simulink model "GS_model"  (R2018b)
settings: Solver=ode5  StartTime=0.0  StopTime=SimuStopTime  FixedStep=T_Simu  RelTol=1e-3
InitFcn:
  | Initial
undefined symbols (not defined in the file or in its folder): Aba10, Aba20, aeroCIP2006_S, aeroCIP2006_X, aeroCIP2006_Y, Agl0, Ass_kS, Ass_n1, Ass_n2, Ass_n3, Ass_n4, Ass_Noise, Ass_R, Ass_Resolution, Ass_TmOrder, AssA_Fix_Abs, AssB_Fix_Abs, AssC_Fix_Abs, AssD_Fix_Abs, AssE_Fix_Aps, AssF_Fix_Aps, C, c_max, c_min, Cd, CenterOfFigNX, CenterOfFigNY, CenterOfFigNZ, CenterOfFigP1, CenterOfFigP2, CenterOfFigPX, CenterOfFigPY, CenterOfFigPZ, Cmu, Crou, DEG2RAD, DiscIntNeverNeededParam, Eg_Dir, Eg_F, Eg_PrepareTime, Eg_r_L_L, Fw_Abf, Fw_Hmax, Fw_J, Fw_Spd0, Fw_Tmax, git_hash_BaseLine, git_hash_Project, Gnss_Noise_Pos, Gnss_Noise_Vel, Gnss_PropgationTime, GyroA_Fix_Abg, GyroA_Noise, GyroB_Fix_Abg, GyroB_Noise, GyroC_Fix_Abg, GyroC_Noise, GyroD_Fix_Abg, GyroD_Noise, h ... (+94)
libraries: simulink x308, sharedutil x46, aerolibutil x37, sharedtransform x31, vrlib x14, aerolibgravity2 x2
(part 8 of 20)

== system GS_model/Subsystem2/Subsystem/Sensor/Magnetometer/MmModel1/Mm_ErrSet ==
  note: TC_MmGNDSet[5*1]
  note: TC_MmErr_Constant[3*1]
  note: TC_MmErr_WildValue[3*1]
  note: TC_MmErr_Jump[5*1]
  note: TC_MmErr_Wave[4*1]
  Mm_MagneticIntensity : Inport
  Mm_Num : Inport  Port=2
  TC_Mm : Inport  Port=3
  Constant1 : Constant  Value=0
  Constant2 : Constant  Value=0
  Demux : Demux  Outputs=[5;3;5;4;3]
  Demux1 : Demux  Outputs=[1;4]
  Demux10 : Demux  Outputs=[1;2]
  Demux6 : Demux  Outputs=[1;2]
  Demux7 : Demux  Outputs=[1;4]
  Demux8 : Demux  Outputs=[1;3]
  Demux9 : Demux  Outputs=[1;3]
  If Action Subsystem3 : Subsystem  TreatAsAtomicUnit=on
  If Action Subsystem4 : Subsystem  TreatAsAtomicUnit=on
  If1 : If  IfExpression=u1 == 1
  Logical Operator{1..5} (5 alike) : Logic  Operator=OR  AllPortsSameDT=off  OutDataTypeStr=boolean
  Merge1 : Merge
  MmErrSet : Subsystem
  Relational Operator{1..10} (10 alike) : RelationalOperator  Operator===  OutDataTypeStr=boolean  RndMeth=Simplest
  Triggered Subsystem5 : Subsystem  TreatAsAtomicUnit=on
  Triggered Subsystem6 : Subsystem  TreatAsAtomicUnit=on
  Triggered Subsystem7 : Subsystem  TreatAsAtomicUnit=on
  Triggered Subsystem8 : Subsystem  TreatAsAtomicUnit=on
  Triggered Subsystem9 : Subsystem  TreatAsAtomicUnit=on
  TM_Mm : Outport
  wires:
  TC_Mm/1 -> Demux/1
  Demux/1 -> Demux1/1
  Demux/2 -> Demux6/1
  Demux/3 -> Demux7/1
  Demux/4 -> Demux9/1
  Demux/5 -> Demux10/1
  Demux1/1 -> Relational Operator1/2, Relational Operator5/2
  Demux1/2 -> Triggered Subsystem6/1(In1)
  Triggered Subsystem6/1(Out1) -> Demux8/1
  Demux8/1 -> If1/1
  If1/1 -> If Action Subsystem4/Action
  Demux8/2 -> If Action Subsystem4/1(In1)
  If Action Subsystem4/1(Out1) -> Merge1/1
  MmErrSet/1(Mm_out) -> If Action Subsystem3/1(In1)
  If1/2 -> If Action Subsystem3/Action
  If Action Subsystem3/1(Out1) -> Merge1/2
  Mm_MagneticIntensity/1 -> MmErrSet/1(Mm_MagneticIntensity)
  Triggered Subsystem9/1(Out1) -> MmErrSet/2(TC_MmErrSet_Constant)
  Triggered Subsystem5/1(Out1) -> MmErrSet/3(TC_MmErrSet_Jump)
  Triggered Subsystem7/1(Out1) -> MmErrSet/4(TC_MmErrSet_Wave)
  Triggered Subsystem8/1(Out1) -> MmErrSet/5(TC_MmErrSet_WildValue)
  Merge1/1 -> TM_Mm/1
  Relational Operator10/1 -> Logical Operator4/1
  Logical Operator4/1 -> Triggered Subsystem8/Enable
  Relational Operator3/1 -> Logical Operator2/1
  Relational Operator6/1 -> Logical Operator1/2
  Demux7/1 -> Relational Operator3/2, Relational Operator7/2
  Mm_Num/1 -> Relational Operator9/1, Relational Operator8/1, Relational Operator7/1, Relational Operator6/1, Relational Operator5/1
  Logical Operator2/1 -> Triggered Subsystem5/Enable
  Relational Operator7/1 -> Logical Operator2/2
  Relational Operator9/1 -> Logical Operator4/2
  Relational Operator4/1 -> Logical Operator3/1
  Logical Operator3/1 -> Triggered Subsystem7/Enable
  Relational Operator8/1 -> Logical Operator3/2
  Demux10/1 -> Relational Operator10/2, Relational Operator9/2
  Relational Operator2/1 -> Logical Operator1/1
  Logical Operator1/1 -> Triggered Subsystem9/Enable
  Demux6/1 -> Relational Operator2/2, Relational Operator6/2
  Constant2/1 -> Relational Operator10/1, Relational Operator4/1, Relational Operator3/1, Relational Operator2/1
  Demux9/1 -> Relational Operator4/2, Relational Operator8/2
  Demux10/2 -> Triggered Subsystem8/1(In1)
  Demux9/2 -> Triggered Subsystem7/1(In1)
  Demux7/2 -> Triggered Subsystem5/1(In1)
  Demux6/2 -> Triggered Subsystem9/1(In1)
  Relational Operator5/1 -> Logical Operator5/2
  Constant1/1 -> Relational Operator1/1
  Relational Operator1/1 -> Logical Operator5/1
  Logical Operator5/1 -> Triggered Subsystem6/Enable

== system GS_model/Subsystem2/Subsystem/Sensor/Magnetometer/MmModel1/Mm_MathModel ==
  Bb : Inport
  Mm_Fix_Abm : Inport  Port=2
  Mm_MtInflunce_Coff : Inport  Port=3
  Mm_Noise : Inport  Port=4
  M_Mt : Inport  Port=5
  Math Function : Math  Operator=transpose  SaturateOnIntegerOverflow=on
  Product1 : Product  Multiplication=Matrix(*)  RndMeth=Zero
  Product2 : Product  Multiplication=Matrix(*)  RndMeth=Zero
  Sum1 : Sum  Inputs=|++
  Sum2 : Sum  Inputs=|++
  Mm_MagneticIntensity : Outport
  wires:
  M_Mt/1 -> Product1/2
  Mm_Noise/1 -> Sum1/2
  Product1/1 -> Sum2/2
  Sum1/1 -> Mm_MagneticIntensity/1
  Mm_Fix_Abm/1 -> Math Function/1
  Mm_MtInflunce_Coff/1 -> Product1/1
  Math Function/1 -> Product2/1
  Bb/1 -> Product2/2
  Sum2/1 -> Sum1/1
  Product2/1 -> Sum2/1

== system GS_model/Subsystem2/Subsystem/Sensor/Magnetometer/MmModel2/Mm_ErrSet ==
  note: TC_MmErr_Wave[4*1]
  note: TC_MmErr_Jump[5*1]
  note: TC_MmErr_WildValue[3*1]
  note: TC_MmErr_Constant[3*1]
  note: TC_MmGNDSet[5*1]
  Mm_MagneticIntensity : Inport
  Mm_Num : Inport  Port=2
  TC_Mm : Inport  Port=3
  Constant1 : Constant  Value=0
  Constant2 : Constant  Value=0
  Demux : Demux  Outputs=[5;3;5;4;3]
  Demux1 : Demux  Outputs=[1;4]
  Demux10 : Demux  Outputs=[1;2]
  Demux6 : Demux  Outputs=[1;2]
  Demux7 : Demux  Outputs=[1;4]
  Demux8 : Demux  Outputs=[1;3]
  Demux9 : Demux  Outputs=[1;3]
  If Action Subsystem3 : Subsystem  TreatAsAtomicUnit=on
  If Action Subsystem4 : Subsystem  TreatAsAtomicUnit=on
  If1 : If  IfExpression=u1 == 1
  Logical Operator{1..5} (5 alike) : Logic  Operator=OR  AllPortsSameDT=off  OutDataTypeStr=boolean
  Merge1 : Merge
  MmErrSet : Subsystem
  Relational Operator{1..10} (10 alike) : RelationalOperator  Operator===  OutDataTypeStr=boolean  RndMeth=Simplest
  Triggered Subsystem5 : Subsystem  TreatAsAtomicUnit=on
  Triggered Subsystem6 : Subsystem  TreatAsAtomicUnit=on
  Triggered Subsystem7 : Subsystem  TreatAsAtomicUnit=on
  Triggered Subsystem8 : Subsystem  TreatAsAtomicUnit=on
  Triggered Subsystem9 : Subsystem  TreatAsAtomicUnit=on
  TM_Mm : Outport
  wires:
  Logical Operator5/1 -> Triggered Subsystem6/Enable
  Relational Operator1/1 -> Logical Operator5/1
  Constant1/1 -> Relational Operator1/1
  Relational Operator5/1 -> Logical Operator5/2
  Demux6/2 -> Triggered Subsystem9/1(In1)
  Demux7/2 -> Triggered Subsystem5/1(In1)
  Demux9/2 -> Triggered Subsystem7/1(In1)
  Demux10/2 -> Triggered Subsystem8/1(In1)
  Demux9/1 -> Relational Operator8/2, Relational Operator4/2
  Constant2/1 -> Relational Operator2/1, Relational Operator3/1, Relational Operator4/1, Relational Operator10/1
  Demux6/1 -> Relational Operator6/2, Relational Operator2/2
  Logical Operator1/1 -> Triggered Subsystem9/Enable
  Relational Operator2/1 -> Logical Operator1/1
  Demux10/1 -> Relational Operator9/2, Relational Operator10/2
  Relational Operator8/1 -> Logical Operator3/2
  Logical Operator3/1 -> Triggered Subsystem7/Enable
  Relational Operator4/1 -> Logical Operator3/1
  Relational Operator9/1 -> Logical Operator4/2
  Relational Operator7/1 -> Logical Operator2/2
  Logical Operator2/1 -> Triggered Subsystem5/Enable
  Mm_Num/1 -> Relational Operator5/1, Relational Operator6/1, Relational Operator7/1, Relational Operator8/1, Relational Operator9/1
  Demux7/1 -> Relational Operator7/2, Relational Operator3/2
  Relational Operator6/1 -> Logical Operator1/2
  Relational Operator3/1 -> Logical Operator2/1
  Logical Operator4/1 -> Triggered Subsystem8/Enable
  Relational Operator10/1 -> Logical Operator4/1
  Merge1/1 -> TM_Mm/1
  Triggered Subsystem8/1(Out1) -> MmErrSet/5(TC_MmErrSet_WildValue)
  Triggered Subsystem7/1(Out1) -> MmErrSet/4(TC_MmErrSet_Wave)
  Triggered Subsystem5/1(Out1) -> MmErrSet/3(TC_MmErrSet_Jump)
  Triggered Subsystem9/1(Out1) -> MmErrSet/2(TC_MmErrSet_Constant)
  Mm_MagneticIntensity/1 -> MmErrSet/1(Mm_MagneticIntensity)
  If Action Subsystem3/1(Out1) -> Merge1/2
  If1/2 -> If Action Subsystem3/Action
  MmErrSet/1(Mm_out) -> If Action Subsystem3/1(In1)
  If Action Subsystem4/1(Out1) -> Merge1/1
  Demux8/2 -> If Action Subsystem4/1(In1)
  If1/1 -> If Action Subsystem4/Action
  Demux8/1 -> If1/1
  Triggered Subsystem6/1(Out1) -> Demux8/1
  Demux1/2 -> Triggered Subsystem6/1(In1)
  Demux1/1 -> Relational Operator5/2, Relational Operator1/2
  Demux/5 -> Demux10/1
  Demux/4 -> Demux9/1
  Demux/3 -> Demux7/1
  Demux/2 -> Demux6/1
  Demux/1 -> Demux1/1
  TC_Mm/1 -> Demux/1

== system GS_model/Subsystem2/Subsystem/Sensor/Magnetometer/MmModel2/Mm_MathModel ==
  Bb : Inport
  Mm_Fix_Abm : Inport  Port=2
  Mm_MtInflunce_Coff : Inport  Port=3
  Mm_Noise : Inport  Port=4
  MtCoff : Inport  Port=5
  Math Function : Math  Operator=transpose  SaturateOnIntegerOverflow=on
  Product1 : Product  Multiplication=Matrix(*)  RndMeth=Zero
  Product2 : Product  Multiplication=Matrix(*)  RndMeth=Zero
  Sum1 : Sum  Inputs=|++
  Sum2 : Sum  Inputs=|++
  Mm_MagneticIntensity : Outport
  wires:
  Product2/1 -> Sum2/1
  Sum2/1 -> Sum1/1
  Bb/1 -> Product2/2
  Math Function/1 -> Product2/1
  Mm_MtInflunce_Coff/1 -> Product1/1
  Mm_Fix_Abm/1 -> Math Function/1
  Sum1/1 -> Mm_MagneticIntensity/1
  Product1/1 -> Sum2/2
  Mm_Noise/1 -> Sum1/2
  MtCoff/1 -> Product1/2

== system GS_model/Subsystem2/Subsystem/Sensor/Magnetometer/MmModel3/Mm_ErrSet ==
  note: TC_MmGNDSet[5*1]
  note: TC_MmErr_Constant[3*1]
  note: TC_MmErr_WildValue[3*1]
  note: TC_MmErr_Jump[5*1]
  note: TC_MmErr_Wave[4*1]
  Mm_MagneticIntensity : Inport
  Mm_Num : Inport  Port=2
  TC_Mm : Inport  Port=3
  Constant1 : Constant  Value=0
  Constant2 : Constant  Value=0
  Demux : Demux  Outputs=[5;3;5;4;3]
  Demux1 : Demux  Outputs=[1;4]
  Demux10 : Demux  Outputs=[1;2]
  Demux6 : Demux  Outputs=[1;2]
  Demux7 : Demux  Outputs=[1;4]
  Demux8 : Demux  Outputs=[1;3]
  Demux9 : Demux  Outputs=[1;3]
  If Action Subsystem3 : Subsystem  TreatAsAtomicUnit=on
  If Action Subsystem4 : Subsystem  TreatAsAtomicUnit=on
  If1 : If  IfExpression=u1 == 1
  Logical Operator{1..5} (5 alike) : Logic  Operator=OR  AllPortsSameDT=off  OutDataTypeStr=boolean
  Merge1 : Merge
  MmErrSet : Subsystem
  Relational Operator{1..10} (10 alike) : RelationalOperator  Operator===  OutDataTypeStr=boolean  RndMeth=Simplest
  Triggered Subsystem5 : Subsystem  TreatAsAtomicUnit=on
  Triggered Subsystem6 : Subsystem  TreatAsAtomicUnit=on
  Triggered Subsystem7 : Subsystem  TreatAsAtomicUnit=on
  Triggered Subsystem8 : Subsystem  TreatAsAtomicUnit=on
  Triggered Subsystem9 : Subsystem  TreatAsAtomicUnit=on
  TM_Mm : Outport
  wires:
  TC_Mm/1 -> Demux/1
  Demux/1 -> Demux1/1
  Demux/2 -> Demux6/1
  Demux/3 -> Demux7/1
  Demux/4 -> Demux9/1
  Demux/5 -> Demux10/1
  Demux1/1 -> Relational Operator1/2, Relational Operator5/2
  Demux1/2 -> Triggered Subsystem6/1(In1)
  Triggered Subsystem6/1(Out1) -> Demux8/1
  Demux8/1 -> If1/1
  If1/1 -> If Action Subsystem4/Action
  Demux8/2 -> If Action Subsystem4/1(In1)
  If Action Subsystem4/1(Out1) -> Merge1/1
  MmErrSet/1(Mm_out) -> If Action Subsystem3/1(In1)
  If1/2 -> If Action Subsystem3/Action
  If Action Subsystem3/1(Out1) -> Merge1/2
  Mm_MagneticIntensity/1 -> MmErrSet/1(Mm_MagneticIntensity)
  Triggered Subsystem9/1(Out1) -> MmErrSet/2(TC_MmErrSet_Constant)
  Triggered Subsystem5/1(Out1) -> MmErrSet/3(TC_MmErrSet_Jump)
  Triggered Subsystem7/1(Out1) -> MmErrSet/4(TC_MmErrSet_Wave)
  Triggered Subsystem8/1(Out1) -> MmErrSet/5(TC_MmErrSet_WildValue)
  Merge1/1 -> TM_Mm/1
  Relational Operator10/1 -> Logical Operator4/1
  Logical Operator4/1 -> Triggered Subsystem8/Enable
  Relational Operator3/1 -> Logical Operator2/1
  Relational Operator6/1 -> Logical Operator1/2
  Demux7/1 -> Relational Operator3/2, Relational Operator7/2
  Mm_Num/1 -> Relational Operator9/1, Relational Operator8/1, Relational Operator7/1, Relational Operator6/1, Relational Operator5/1
  Logical Operator2/1 -> Triggered Subsystem5/Enable
  Relational Operator7/1 -> Logical Operator2/2
  Relational Operator9/1 -> Logical Operator4/2
  Relational Operator4/1 -> Logical Operator3/1
  Logical Operator3/1 -> Triggered Subsystem7/Enable
  Relational Operator8/1 -> Logical Operator3/2
  Demux10/1 -> Relational Operator10/2, Relational Operator9/2
  Relational Operator2/1 -> Logical Operator1/1
  Logical Operator1/1 -> Triggered Subsystem9/Enable
  Demux6/1 -> Relational Operator2/2, Relational Operator6/2
  Constant2/1 -> Relational Operator10/1, Relational Operator4/1, Relational Operator3/1, Relational Operator2/1
  Demux9/1 -> Relational Operator4/2, Relational Operator8/2
  Demux10/2 -> Triggered Subsystem8/1(In1)
  Demux9/2 -> Triggered Subsystem7/1(In1)
  Demux7/2 -> Triggered Subsystem5/1(In1)
  Demux6/2 -> Triggered Subsystem9/1(In1)
  Relational Operator5/1 -> Logical Operator5/2
  Constant1/1 -> Relational Operator1/1
  Relational Operator1/1 -> Logical Operator5/1
  Logical Operator5/1 -> Triggered Subsystem6/Enable

== system GS_model/Subsystem2/Subsystem/Sensor/Magnetometer/MmModel3/Mm_MathModel ==
  Bb : Inport
  Mm_Fix_Abm : Inport  Port=2
  Mm_MtInflunce_Coff : Inport  Port=3
  Mm_Noise : Inport  Port=4
  MtCoff : Inport  Port=5
  Math Function : Math  Operator=transpose  SaturateOnIntegerOverflow=on
  Product1 : Product  Multiplication=Matrix(*)  RndMeth=Zero
  Product2 : Product  Multiplication=Matrix(*)  RndMeth=Zero
  Sum1 : Sum  Inputs=|++
  Sum2 : Sum  Inputs=|++
  Mm_MagneticIntensity : Outport
  wires:
  MtCoff/1 -> Product1/2
  Mm_Noise/1 -> Sum1/2
  Product1/1 -> Sum2/2
  Sum1/1 -> Mm_MagneticIntensity/1
  Mm_Fix_Abm/1 -> Math Function/1
  Mm_MtInflunce_Coff/1 -> Product1/1
  Math Function/1 -> Product2/1
  Bb/1 -> Product2/2
  Sum2/1 -> Sum1/1
  Product2/1 -> Sum2/1

== system GS_model/Subsystem2/Subsystem/Sensor/Magnetometer/MmModel4/Mm_ErrSet ==
  note: TC_MmErr_Wave[4*1]
  note: TC_MmErr_Jump[5*1]
  note: TC_MmErr_WildValue[3*1]
  note: TC_MmErr_Constant[3*1]
  note: TC_MmGNDSet[5*1]
  Mm_MagneticIntensity : Inport
  Mm_Num : Inport  Port=2
  TC_Mm : Inport  Port=3
  Constant1 : Constant  Value=0
  Constant2 : Constant  Value=0
  Demux : Demux  Outputs=[5;3;5;4;3]
  Demux1 : Demux  Outputs=[1;4]
  Demux10 : Demux  Outputs=[1;2]
  Demux6 : Demux  Outputs=[1;2]
  Demux7 : Demux  Outputs=[1;4]
  Demux8 : Demux  Outputs=[1;3]
  Demux9 : Demux  Outputs=[1;3]
  If Action Subsystem3 : Subsystem  TreatAsAtomicUnit=on
  If Action Subsystem4 : Subsystem  TreatAsAtomicUnit=on
  If1 : If  IfExpression=u1 == 1
  Logical Operator{1..5} (5 alike) : Logic  Operator=OR  AllPortsSameDT=off  OutDataTypeStr=boolean
  Merge1 : Merge
  MmErrSet : Subsystem
  Relational Operator{1..10} (10 alike) : RelationalOperator  Operator===  OutDataTypeStr=boolean  RndMeth=Simplest
  Triggered Subsystem5 : Subsystem  TreatAsAtomicUnit=on
  Triggered Subsystem6 : Subsystem  TreatAsAtomicUnit=on
  Triggered Subsystem7 : Subsystem  TreatAsAtomicUnit=on
  Triggered Subsystem8 : Subsystem  TreatAsAtomicUnit=on
  Triggered Subsystem9 : Subsystem  TreatAsAtomicUnit=on
  TM_Mm : Outport
  wires:
  Logical Operator5/1 -> Triggered Subsystem6/Enable
  Relational Operator1/1 -> Logical Operator5/1
  Constant1/1 -> Relational Operator1/1
  Relational Operator5/1 -> Logical Operator5/2
  Demux6/2 -> Triggered Subsystem9/1(In1)
  Demux7/2 -> Triggered Subsystem5/1(In1)
  Demux9/2 -> Triggered Subsystem7/1(In1)
  Demux10/2 -> Triggered Subsystem8/1(In1)
  Demux9/1 -> Relational Operator8/2, Relational Operator4/2
  Constant2/1 -> Relational Operator2/1, Relational Operator3/1, Relational Operator4/1, Relational Operator10/1
  Demux6/1 -> Relational Operator6/2, Relational Operator2/2
  Logical Operator1/1 -> Triggered Subsystem9/Enable
  Relational Operator2/1 -> Logical Operator1/1
  Demux10/1 -> Relational Operator9/2, Relational Operator10/2
  Relational Operator8/1 -> Logical Operator3/2
  Logical Operator3/1 -> Triggered Subsystem7/Enable
  Relational Operator4/1 -> Logical Operator3/1
  Relational Operator9/1 -> Logical Operator4/2
  Relational Operator7/1 -> Logical Operator2/2
  Logical Operator2/1 -> Triggered Subsystem5/Enable
  Mm_Num/1 -> Relational Operator5/1, Relational Operator6/1, Relational Operator7/1, Relational Operator8/1, Relational Operator9/1
  Demux7/1 -> Relational Operator7/2, Relational Operator3/2
  Relational Operator6/1 -> Logical Operator1/2
  Relational Operator3/1 -> Logical Operator2/1
  Logical Operator4/1 -> Triggered Subsystem8/Enable
  Relational Operator10/1 -> Logical Operator4/1
  Merge1/1 -> TM_Mm/1
  Triggered Subsystem8/1(Out1) -> MmErrSet/5(TC_MmErrSet_WildValue)
  Triggered Subsystem7/1(Out1) -> MmErrSet/4(TC_MmErrSet_Wave)
  Triggered Subsystem5/1(Out1) -> MmErrSet/3(TC_MmErrSet_Jump)
  Triggered Subsystem9/1(Out1) -> MmErrSet/2(TC_MmErrSet_Constant)
  Mm_MagneticIntensity/1 -> MmErrSet/1(Mm_MagneticIntensity)
  If Action Subsystem3/1(Out1) -> Merge1/2
  If1/2 -> If Action Subsystem3/Action
  MmErrSet/1(Mm_out) -> If Action Subsystem3/1(In1)
  If Action Subsystem4/1(Out1) -> Merge1/1
  Demux8/2 -> If Action Subsystem4/1(In1)
  If1/1 -> If Action Subsystem4/Action
  Demux8/1 -> If1/1
  Triggered Subsystem6/1(Out1) -> Demux8/1
  Demux1/2 -> Triggered Subsystem6/1(In1)
  Demux1/1 -> Relational Operator5/2, Relational Operator1/2
  Demux/5 -> Demux10/1
  Demux/4 -> Demux9/1
  Demux/3 -> Demux7/1
  Demux/2 -> Demux6/1
  Demux/1 -> Demux1/1
  TC_Mm/1 -> Demux/1

== system GS_model/Subsystem2/Subsystem/Sensor/Magnetometer/MmModel4/Mm_MathModel ==
  Bb : Inport
  Mm_Fix_Abm : Inport  Port=2
  Mm_MtInflunce_Coff : Inport  Port=3
  Mm_Noise : Inport  Port=4
  MtCoff : Inport  Port=5
  Math Function : Math  Operator=transpose  SaturateOnIntegerOverflow=on
  Product1 : Product  Multiplication=Matrix(*)  RndMeth=Zero
  Product2 : Product  Multiplication=Matrix(*)  RndMeth=Zero
  Sum1 : Sum  Inputs=|++
  Sum2 : Sum  Inputs=|++
  Mm_MagneticIntensity : Outport
  wires:
  Product2/1 -> Sum2/1
  Sum2/1 -> Sum1/1
  Bb/1 -> Product2/2
  Math Function/1 -> Product2/1
  Mm_MtInflunce_Coff/1 -> Product1/1
  Mm_Fix_Abm/1 -> Math Function/1
  Sum1/1 -> Mm_MagneticIntensity/1
  Product1/1 -> Sum2/2
  Mm_Noise/1 -> Sum1/2
  MtCoff/1 -> Product1/2

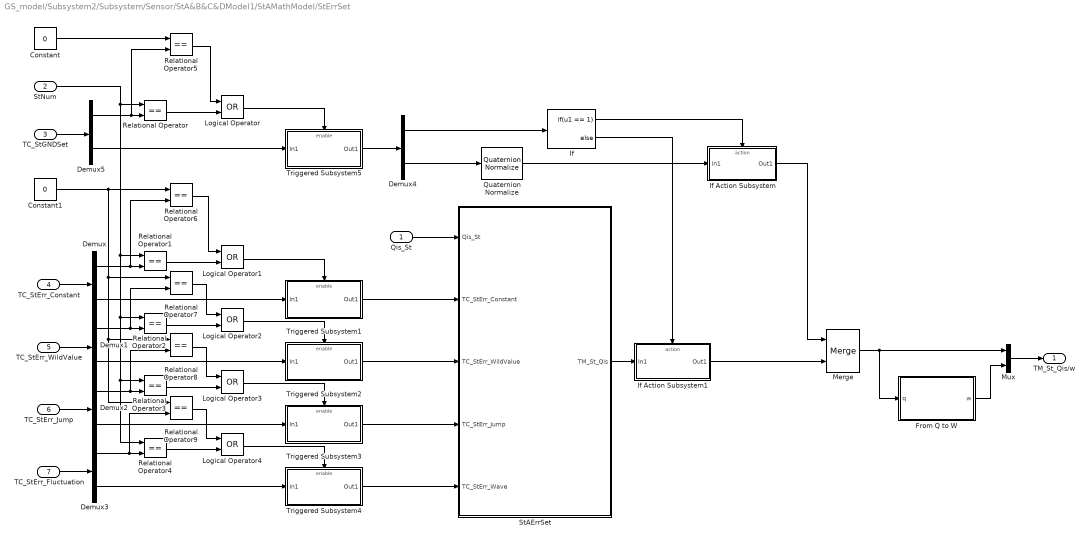
== system GS_model/Subsystem2/Subsystem/Sensor/StA&B&C&DModel1/StAMathModel/StErrSet ==
  Qis_St : Inport
  StNum : Inport  Port=2
  TC_StGNDSet : Inport  Port=3
  TC_StErr_Constant : Inport  Port=4
  TC_StErr_WildValue : Inport  Port=5
  TC_StErr_Jump : Inport  Port=6
  TC_StErr_Fluctuation : Inport  Port=7
  Constant : Constant  Value=0
  Constant1 : Constant  Value=0
  Demux : Demux  Outputs=2
  Demux1 : Demux  Outputs=2
  Demux2 : Demux  Outputs=[1;3]
  Demux3 : Demux  Outputs=[1;2]
  Demux4 : Demux  Outputs=[1;4]
  Demux5 : Demux  Outputs=[1;5]
  From Q to W : Subsystem
  If : If  IfExpression=u1 == 1
  If Action Subsystem : Subsystem  TreatAsAtomicUnit=on
  If Action Subsystem1 : Subsystem  TreatAsAtomicUnit=on
  Logical Operator{,1..4} (5 alike) : Logic  Operator=OR  AllPortsSameDT=off  OutDataTypeStr=boolean
  Merge : Merge
  Mux : Mux  Inputs=2
  Quaternion Normalize : sharedutil/Quaternion Normalize  aMode=aMode
      settings: SourceProductBaseCode=AE,PW,MT,VE,VP
  Relational Operator{,1..9} (10 alike) : RelationalOperator  Operator===  OutDataTypeStr=boolean  RndMeth=Simplest
  StAErrSet : Subsystem
  Triggered Subsystem1 : Subsystem  TreatAsAtomicUnit=on
  Triggered Subsystem2 : Subsystem  TreatAsAtomicUnit=on
  Triggered Subsystem3 : Subsystem  TreatAsAtomicUnit=on
  Triggered Subsystem4 : Subsystem  TreatAsAtomicUnit=on
  Triggered Subsystem5 : Subsystem  TreatAsAtomicUnit=on
  TM_St_Qis/w : Outport
  wires:
  Demux/2 -> Triggered Subsystem1/1(In1)
  Demux1/1 -> Relational Operator7/2, Relational Operator2/2
  Demux1/2 -> Triggered Subsystem2/1(In1)
  Demux2/1 -> Relational Operator8/2, Relational Operator3/2
  Demux3/1 -> Relational Operator9/2, Relational Operator4/2
  Demux3/2 -> Triggered Subsystem4/1(In1)
  TC_StErr_Constant/1 -> Demux/1
  TC_StErr_WildValue/1 -> Demux1/1
  TC_StErr_Fluctuation/1 -> Demux3/1
  Triggered Subsystem1/1(Out1) -> StAErrSet/2(TC_StErr_Constant)
  Triggered Subsystem2/1(Out1) -> StAErrSet/3(TC_StErr_WildValue)
  Triggered Subsystem3/1(Out1) -> StAErrSet/4(TC_StErr_Jump)
  Triggered Subsystem4/1(Out1) -> StAErrSet/5(TC_StErr_Wave)
  Demux4/1 -> If/1
  If/1 -> If Action Subsystem/Action
  Demux4/2 -> Quaternion Normalize/1
  If/2 -> If Action Subsystem1/Action
  StAErrSet/1(TM_St_Qis) -> If Action Subsystem1/1(In1)
  If Action Subsystem/1(Out1) -> Merge/1
  If Action Subsystem1/1(Out1) -> Merge/2
  Demux2/2 -> Triggered Subsystem3/1(In1)
  TC_StErr_Jump/1 -> Demux2/1
  Triggered Subsystem5/1(Out1) -> Demux4/1
  TC_StGNDSet/1 -> Demux5/1
  StNum/1 -> Relational Operator4/1, Relational Operator3/1, Relational Operator2/1, Relational Operator1/1, Relational Operator/1
  Relational Operator5/1 -> Logical Operator/1
  Demux5/1 -> Relational Operator5/2, Relational Operator/2
  Constant/1 -> Relational Operator5/1
  Relational Operator/1 -> Logical Operator/2
  Logical Operator/1 -> Triggered Subsystem5/Enable
  Relational Operator6/1 -> Logical Operator1/1
  Constant1/1 -> Relational Operator9/1, Relational Operator8/1, Relational Operator7/1, Relational Operator6/1
  Demux/1 -> Relational Operator6/2, Relational Operator1/2
  Relational Operator1/1 -> Logical Operator1/2
  Logical Operator1/1 -> Triggered Subsystem1/Enable
  Relational Operator2/1 -> Logical Operator2/2
  Logical Operator2/1 -> Triggered Subsystem2/Enable
  Relational Operator7/1 -> Logical Operator2/1
  Relational Operator3/1 -> Logical Operator3/2
  Logical Operator3/1 -> Triggered Subsystem3/Enable
  Relational Operator8/1 -> Logical Operator3/1
  Logical Operator4/1 -> Triggered Subsystem4/Enable
  Relational Operator4/1 -> Logical Operator4/2
  Relational Operator9/1 -> Logical Operator4/1
  Demux5/2 -> Triggered Subsystem5/1(In1)
  Quaternion Normalize/1 -> If Action Subsystem/1(In1)
  Merge/1 -> From Q to W/1(q), Mux/1
  From Q to W/1(w) -> Mux/2
  Mux/1 -> TM_St_Qis/w/1
  Qis_St/1 -> StAErrSet/1(Qis_St)

== system GS_model/Subsystem2/Subsystem/Sensor/StA&B&C&DModel1/StAMathModel/StMathModel ==
  note: Qbs_St
  Qib : Inport
  Cons_StNoise : Inport  Port=2
  Qsb_StFix : Inport  Port=3
  TC_StFixErr : Inport  Port=4
  TC_StNoiseCoff : Inport  Port=5
  StNum : Inport  Port=6
  3 : Subsystem
  Constant : Constant  Value=0
  Constant1 : Constant  Value=0
  Demux : Demux  Outputs=[1;4]
  Demux1 : Demux  Outputs=2
  Logical Operator : Logic  Operator=OR  AllPortsSameDT=off  OutDataTypeStr=boolean
  Logical Operator1 : Logic  Operator=OR  AllPortsSameDT=off  OutDataTypeStr=boolean
  Quaternion Inverse : aerolibutil/Quaternion Inverse
  Quaternion Multiplication : aerolibutil/Quaternion Multiplication
  Quaternion Multiplication2 : aerolibutil/Quaternion Multiplication
  Quaternion Multiplication4 : aerolibutil/Quaternion Multiplication
  Quaternion Normalize : sharedutil/Quaternion Normalize  aMode=aMode
      settings: SourceProductBaseCode=AE,PW,MT,VE,VP
  Quaternion Normalize2 : sharedutil/Quaternion Normalize  aMode=aMode
      settings: SourceProductBaseCode=AE,PW,MT,VE,VP
  Relational Operator{,1..3} (4 alike) : RelationalOperator  Operator===  OutDataTypeStr=boolean  RndMeth=Simplest
  Triggered Subsystem1 : Subsystem  TreatAsAtomicUnit=on
  Triggered Subsystem2 : Subsystem  TreatAsAtomicUnit=on
  Qis_St : Outport
  wires:
  Triggered Subsystem2/1(Out1) -> 3/1(TC_StNoiseCoff)
  Demux/2 -> Triggered Subsystem1/1(In1)
  Triggered Subsystem1/1(Out1) -> Quaternion Normalize2/1
  Quaternion Normalize/1 -> Quaternion Multiplication/1
  Demux1/1 -> Relational Operator3/2, Relational Operator/2
  Demux1/2 -> Triggered Subsystem2/1(In1)
  Demux/1 -> Relational Operator2/2, Relational Operator1/2
  Quaternion Multiplication2/1 -> Quaternion Multiplication4/1
  TC_StNoiseCoff/1 -> Demux1/1
  Quaternion Normalize2/1 -> Quaternion Multiplication/2
  3/1(Q_StNoise) -> Quaternion Multiplication4/2
  Quaternion Multiplication/1 -> Quaternion Inverse/1
  Qib/1 -> Quaternion Multiplication2/1
  Qsb_StFix/1 -> Quaternion Normalize/1
  TC_StFixErr/1 -> Demux/1
  Quaternion Multiplication4/1 -> Qis_St/1
  Cons_StNoise/1 -> 3/2(Cons_StNoise)
  StNum/1 -> Relational Operator/1, Relational Operator1/1
  Relational Operator1/1 -> Logical Operator/2
  Constant/1 -> Relational Operator2/1
  Relational Operator2/1 -> Logical Operator/1
  Logical Operator/1 -> Triggered Subsystem1/Enable
  Relational Operator/1 -> Logical Operator1/2
  Constant1/1 -> Relational Operator3/1
  Relational Operator3/1 -> Logical Operator1/1
  Logical Operator1/1 -> Triggered Subsystem2/Enable
  Quaternion Inverse/1 -> Quaternion Multiplication2/2

== system GS_model/Subsystem2/Subsystem/Sensor/StA&B&C&DModel1/StAMathModel/Subsystem ==
  note: 0-自主
      | 1-常有效
      | 2-常无效
  Sun_b : Inport
  Sunshine : Inport  Port=2
  Tc_ValidSet : Inport  Port=3
  Qsb_StAFix : Inport  Port=4
  SEA : Inport  Port=5
  EEA : Inport  Port=6
  Qob : Inport  Port=7
  Qis : Inport  Port=8
  StNum : Inport  Port=9
  Constant1 : Constant  Value=0
  Constant2 : Constant  Value=[1;0;0;0]
  Constant3 : Constant
  Constant4 : Constant  Value=0
  Demux1 : Demux  Outputs=2
  Logical Operator1 : Logic  Operator=OR  AllPortsSameDT=off  OutDataTypeStr=boolean
  Relational Operator : RelationalOperator  Operator===  OutDataTypeStr=boolean  RndMeth=Simplest
  Relational Operator3 : RelationalOperator  Operator===  OutDataTypeStr=boolean  RndMeth=Simplest
  Subsystem : Subsystem
  Switch : Switch  Criteria=u2 > Threshold  Threshold=0.5
  Switch1 : Switch  Criteria=u2 > Threshold  Threshold=0.5
  Switch2 : Switch  Criteria=u2 > Threshold  Threshold=1.5
  Triggered Subsystem2 : Subsystem  TreatAsAtomicUnit=on
  Agl_St&SunEarth : Outport
  Valid : Outport  Port=2
  Qis_St : Outport  Port=3
  wires:
  Switch/1 -> Qis_St/1
  Switch2/1 -> Valid/1, Switch/2
  Sun_b/1 -> Subsystem/1(Sun_b)
  Sunshine/1 -> Subsystem/2(Sunshine)
  Qsb_StAFix/1 -> Subsystem/3(Qsb_StAFix)
  SEA/1 -> Subsystem/4(SEA)
  EEA/1 -> Subsystem/5(EEA)
  Qob/1 -> Subsystem/6(Qob)
  Subsystem/2(Agl_St&SunEarth) -> Agl_St&SunEarth/1
  Relational Operator3/1 -> Logical Operator1/1
  Relational Operator/1 -> Logical Operator1/2
  Constant1/1 -> Relational Operator3/1
  Demux1/2 -> Triggered Subsystem2/1(In1)
  StNum/1 -> Relational Operator/1
  Demux1/1 -> Relational Operator3/2, Relational Operator/2
  Tc_ValidSet/1 -> Demux1/1
  Triggered Subsystem2/1(Out1) -> Switch1/2, Switch2/2
  Subsystem/1(Valid) -> Switch1/3
  Constant3/1 -> Switch1/1
  Switch1/1 -> Switch2/3
  Constant4/1 -> Switch2/1
  Logical Operator1/1 -> Triggered Subsystem2/Enable
  Qis/1 -> Switch/1
  Constant2/1 -> Switch/3

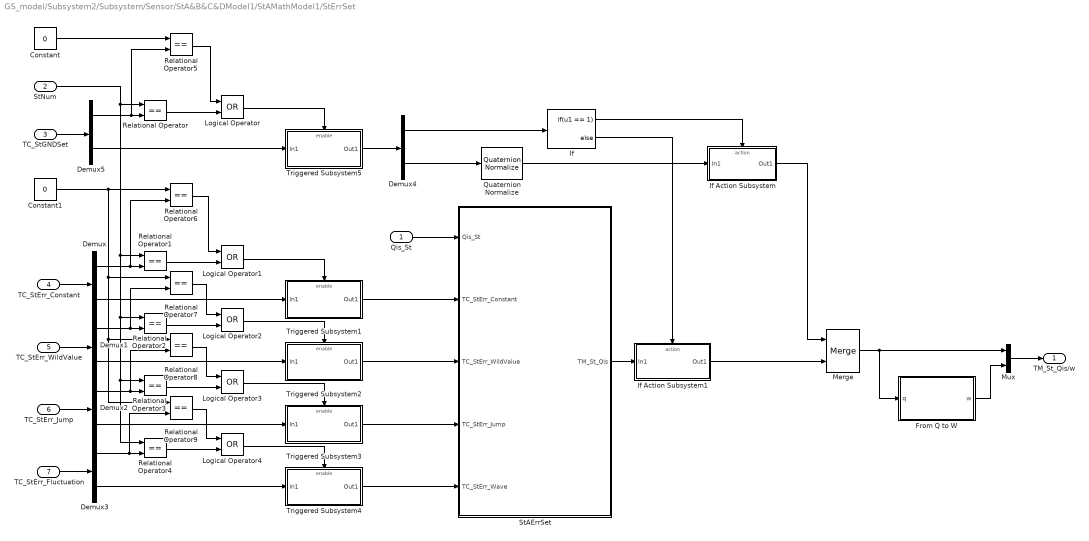
== system GS_model/Subsystem2/Subsystem/Sensor/StA&B&C&DModel1/StAMathModel1/StErrSet ==
  Qis_St : Inport
  StNum : Inport  Port=2
  TC_StGNDSet : Inport  Port=3
  TC_StErr_Constant : Inport  Port=4
  TC_StErr_WildValue : Inport  Port=5
  TC_StErr_Jump : Inport  Port=6
  TC_StErr_Fluctuation : Inport  Port=7
  Constant : Constant  Value=0
  Constant1 : Constant  Value=0
  Demux : Demux  Outputs=2
  Demux1 : Demux  Outputs=2
  Demux2 : Demux  Outputs=[1;3]
  Demux3 : Demux  Outputs=[1;2]
  Demux4 : Demux  Outputs=[1;4]
  Demux5 : Demux  Outputs=[1;5]
  From Q to W : Subsystem
  If : If  IfExpression=u1 == 1
  If Action Subsystem : Subsystem  TreatAsAtomicUnit=on
  If Action Subsystem1 : Subsystem  TreatAsAtomicUnit=on
  Logical Operator{,1..4} (5 alike) : Logic  Operator=OR  AllPortsSameDT=off  OutDataTypeStr=boolean
  Merge : Merge
  Mux : Mux  Inputs=2
  Quaternion Normalize : sharedutil/Quaternion Normalize  aMode=aMode
      settings: SourceProductBaseCode=AE,PW,MT,VE,VP
  Relational Operator{,1..9} (10 alike) : RelationalOperator  Operator===  OutDataTypeStr=boolean  RndMeth=Simplest
  StAErrSet : Subsystem
  Triggered Subsystem1 : Subsystem  TreatAsAtomicUnit=on
  Triggered Subsystem2 : Subsystem  TreatAsAtomicUnit=on
  Triggered Subsystem3 : Subsystem  TreatAsAtomicUnit=on
  Triggered Subsystem4 : Subsystem  TreatAsAtomicUnit=on
  Triggered Subsystem5 : Subsystem  TreatAsAtomicUnit=on
  TM_St_Qis/w : Outport
  wires:
  Qis_St/1 -> StAErrSet/1(Qis_St)
  Mux/1 -> TM_St_Qis/w/1
  From Q to W/1(w) -> Mux/2
  Merge/1 -> Mux/1, From Q to W/1(q)
  Quaternion Normalize/1 -> If Action Subsystem/1(In1)
  Demux5/2 -> Triggered Subsystem5/1(In1)
  Relational Operator9/1 -> Logical Operator4/1
  Relational Operator4/1 -> Logical Operator4/2
  Logical Operator4/1 -> Triggered Subsystem4/Enable
  Relational Operator8/1 -> Logical Operator3/1
  Logical Operator3/1 -> Triggered Subsystem3/Enable
  Relational Operator3/1 -> Logical Operator3/2
  Relational Operator7/1 -> Logical Operator2/1
  Logical Operator2/1 -> Triggered Subsystem2/Enable
  Relational Operator2/1 -> Logical Operator2/2
  Logical Operator1/1 -> Triggered Subsystem1/Enable
  Relational Operator1/1 -> Logical Operator1/2
  Demux/1 -> Relational Operator1/2, Relational Operator6/2
  Constant1/1 -> Relational Operator6/1, Relational Operator7/1, Relational Operator8/1, Relational Operator9/1
  Relational Operator6/1 -> Logical Operator1/1
  Logical Operator/1 -> Triggered Subsystem5/Enable
  Relational Operator/1 -> Logical Operator/2
  Constant/1 -> Relational Operator5/1
  Demux5/1 -> Relational Operator/2, Relational Operator5/2
  Relational Operator5/1 -> Logical Operator/1
  StNum/1 -> Relational Operator/1, Relational Operator1/1, Relational Operator2/1, Relational Operator3/1, Relational Operator4/1
  TC_StGNDSet/1 -> Demux5/1
  Triggered Subsystem5/1(Out1) -> Demux4/1
  TC_StErr_Jump/1 -> Demux2/1
  Demux2/2 -> Triggered Subsystem3/1(In1)
  If Action Subsystem1/1(Out1) -> Merge/2
  If Action Subsystem/1(Out1) -> Merge/1
  StAErrSet/1(TM_St_Qis) -> If Action Subsystem1/1(In1)
  If/2 -> If Action Subsystem1/Action
  Demux4/2 -> Quaternion Normalize/1
  If/1 -> If Action Subsystem/Action
  Demux4/1 -> If/1
  Triggered Subsystem4/1(Out1) -> StAErrSet/5(TC_StErr_Wave)
  Triggered Subsystem3/1(Out1) -> StAErrSet/4(TC_StErr_Jump)
  Triggered Subsystem2/1(Out1) -> StAErrSet/3(TC_StErr_WildValue)
  Triggered Subsystem1/1(Out1) -> StAErrSet/2(TC_StErr_Constant)
  TC_StErr_Fluctuation/1 -> Demux3/1
  TC_StErr_WildValue/1 -> Demux1/1
  TC_StErr_Constant/1 -> Demux/1
  Demux3/2 -> Triggered Subsystem4/1(In1)
  Demux3/1 -> Relational Operator4/2, Relational Operator9/2
  Demux2/1 -> Relational Operator3/2, Relational Operator8/2
  Demux1/2 -> Triggered Subsystem2/1(In1)
  Demux1/1 -> Relational Operator2/2, Relational Operator7/2
  Demux/2 -> Triggered Subsystem1/1(In1)

== system GS_model/Subsystem2/Subsystem/Sensor/StA&B&C&DModel1/StAMathModel1/StMathModel ==
  note: Qbs_St
  Qib : Inport
  Cons_StNoise : Inport  Port=2
  Qsb_StFix : Inport  Port=3
  TC_StFixErr : Inport  Port=4
  TC_StNoiseCoff : Inport  Port=5
  StNum : Inport  Port=6
  3 : Subsystem
  Constant : Constant  Value=0
  Constant1 : Constant  Value=0
  Demux : Demux  Outputs=[1;4]
  Demux1 : Demux  Outputs=2
  Logical Operator : Logic  Operator=OR  AllPortsSameDT=off  OutDataTypeStr=boolean
  Logical Operator1 : Logic  Operator=OR  AllPortsSameDT=off  OutDataTypeStr=boolean
  Quaternion Inverse : aerolibutil/Quaternion Inverse
  Quaternion Multiplication : aerolibutil/Quaternion Multiplication
  Quaternion Multiplication2 : aerolibutil/Quaternion Multiplication
  Quaternion Multiplication4 : aerolibutil/Quaternion Multiplication
  Quaternion Normalize : sharedutil/Quaternion Normalize  aMode=aMode
      settings: SourceProductBaseCode=AE,PW,MT,VE,VP
  Quaternion Normalize2 : sharedutil/Quaternion Normalize  aMode=aMode
      settings: SourceProductBaseCode=AE,PW,MT,VE,VP
  Relational Operator{,1..3} (4 alike) : RelationalOperator  Operator===  OutDataTypeStr=boolean  RndMeth=Simplest
  Triggered Subsystem1 : Subsystem  TreatAsAtomicUnit=on
  Triggered Subsystem2 : Subsystem  TreatAsAtomicUnit=on
  Qis_St : Outport
  wires:
  Quaternion Inverse/1 -> Quaternion Multiplication2/2
  Logical Operator1/1 -> Triggered Subsystem2/Enable
  Relational Operator3/1 -> Logical Operator1/1
  Constant1/1 -> Relational Operator3/1
  Relational Operator/1 -> Logical Operator1/2
  Logical Operator/1 -> Triggered Subsystem1/Enable
  Relational Operator2/1 -> Logical Operator/1
  Constant/1 -> Relational Operator2/1
  Relational Operator1/1 -> Logical Operator/2
  StNum/1 -> Relational Operator1/1, Relational Operator/1
  Cons_StNoise/1 -> 3/2(Cons_StNoise)
  Quaternion Multiplication4/1 -> Qis_St/1
  TC_StFixErr/1 -> Demux/1
  Qsb_StFix/1 -> Quaternion Normalize/1
  Qib/1 -> Quaternion Multiplication2/1
  Quaternion Multiplication/1 -> Quaternion Inverse/1
  3/1(Q_StNoise) -> Quaternion Multiplication4/2
  Quaternion Normalize2/1 -> Quaternion Multiplication/2
  TC_StNoiseCoff/1 -> Demux1/1
  Quaternion Multiplication2/1 -> Quaternion Multiplication4/1
  Demux/1 -> Relational Operator1/2, Relational Operator2/2
  Demux1/2 -> Triggered Subsystem2/1(In1)
  Demux1/1 -> Relational Operator/2, Relational Operator3/2
  Quaternion Normalize/1 -> Quaternion Multiplication/1
  Triggered Subsystem1/1(Out1) -> Quaternion Normalize2/1
  Demux/2 -> Triggered Subsystem1/1(In1)
  Triggered Subsystem2/1(Out1) -> 3/1(TC_StNoiseCoff)

== system GS_model/Subsystem2/Subsystem/Sensor/StA&B&C&DModel1/StAMathModel1/Subsystem ==
  note: 0-自主
      | 1-常有效
      | 2-常无效
  Sun_b : Inport
  Sunshine : Inport  Port=2
  Tc_ValidSet : Inport  Port=3
  Qsb_StAFix : Inport  Port=4
  SEA : Inport  Port=5
  EEA : Inport  Port=6
  Qob : Inport  Port=7
  Qis : Inport  Port=8
  StNum : Inport  Port=9
  Constant1 : Constant  Value=0
  Constant2 : Constant  Value=[1;0;0;0]
  Constant3 : Constant
  Constant4 : Constant  Value=0
  Demux1 : Demux  Outputs=2
  Logical Operator1 : Logic  Operator=OR  AllPortsSameDT=off  OutDataTypeStr=boolean
  Relational Operator : RelationalOperator  Operator===  OutDataTypeStr=boolean  RndMeth=Simplest
  Relational Operator3 : RelationalOperator  Operator===  OutDataTypeStr=boolean  RndMeth=Simplest
  Subsystem : Subsystem
  Switch : Switch  Criteria=u2 > Threshold  Threshold=0.5
  Switch1 : Switch  Criteria=u2 > Threshold  Threshold=0.5
  Switch2 : Switch  Criteria=u2 > Threshold  Threshold=1.5
  Triggered Subsystem2 : Subsystem  TreatAsAtomicUnit=on
  Agl_St&SunEarth : Outport
  Valid : Outport  Port=2
  Qis_St : Outport  Port=3
  wires:
  Constant2/1 -> Switch/3
  Qis/1 -> Switch/1
  Logical Operator1/1 -> Triggered Subsystem2/Enable
  Constant4/1 -> Switch2/1
  Switch1/1 -> Switch2/3
  Constant3/1 -> Switch1/1
  Subsystem/1(Valid) -> Switch1/3
  Triggered Subsystem2/1(Out1) -> Switch2/2, Switch1/2
  Tc_ValidSet/1 -> Demux1/1
  Demux1/1 -> Relational Operator/2, Relational Operator3/2
  StNum/1 -> Relational Operator/1
  Demux1/2 -> Triggered Subsystem2/1(In1)
  Constant1/1 -> Relational Operator3/1
  Relational Operator/1 -> Logical Operator1/2
  Relational Operator3/1 -> Logical Operator1/1
  Subsystem/2(Agl_St&SunEarth) -> Agl_St&SunEarth/1
  Qob/1 -> Subsystem/6(Qob)
  EEA/1 -> Subsystem/5(EEA)
  SEA/1 -> Subsystem/4(SEA)
  Qsb_StAFix/1 -> Subsystem/3(Qsb_StAFix)
  Sunshine/1 -> Subsystem/2(Sunshine)
  Sun_b/1 -> Subsystem/1(Sun_b)
  Switch2/1 -> Switch/2, Valid/1
  Switch/1 -> Qis_St/1

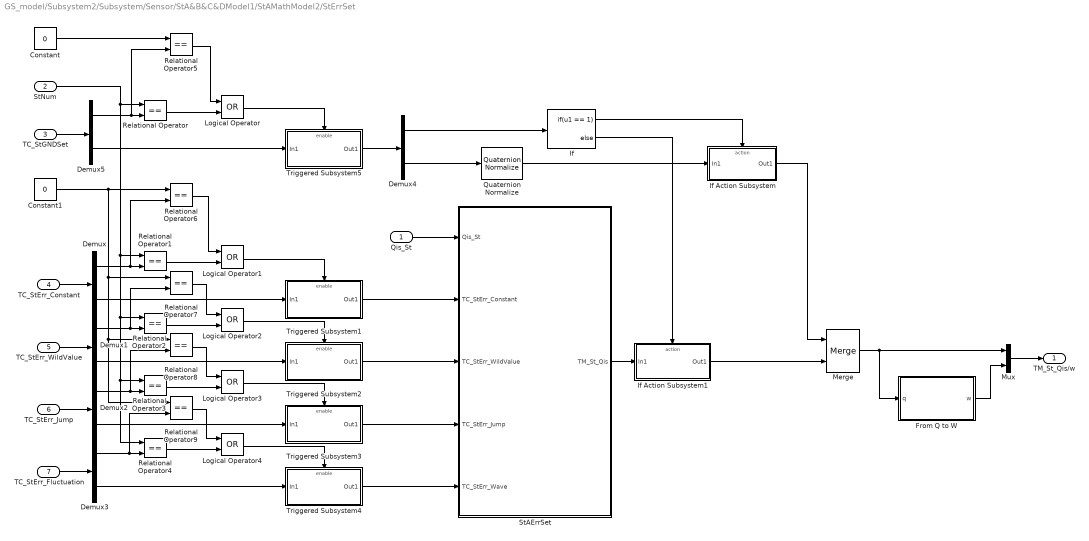
== system GS_model/Subsystem2/Subsystem/Sensor/StA&B&C&DModel1/StAMathModel2/StErrSet ==
  Qis_St : Inport
  StNum : Inport  Port=2
  TC_StGNDSet : Inport  Port=3
  TC_StErr_Constant : Inport  Port=4
  TC_StErr_WildValue : Inport  Port=5
  TC_StErr_Jump : Inport  Port=6
  TC_StErr_Fluctuation : Inport  Port=7
  Constant : Constant  Value=0
  Constant1 : Constant  Value=0
  Demux : Demux  Outputs=2
  Demux1 : Demux  Outputs=2
  Demux2 : Demux  Outputs=[1;3]
  Demux3 : Demux  Outputs=[1;2]
  Demux4 : Demux  Outputs=[1;4]
  Demux5 : Demux  Outputs=[1;5]
  From Q to W : Subsystem
  If : If  IfExpression=u1 == 1
  If Action Subsystem : Subsystem  TreatAsAtomicUnit=on
  If Action Subsystem1 : Subsystem  TreatAsAtomicUnit=on
  Logical Operator{,1..4} (5 alike) : Logic  Operator=OR  AllPortsSameDT=off  OutDataTypeStr=boolean
  Merge : Merge
  Mux : Mux  Inputs=2
  Quaternion Normalize : sharedutil/Quaternion Normalize  aMode=aMode
      settings: SourceProductBaseCode=AE,PW,MT,VE,VP
  Relational Operator{,1..9} (10 alike) : RelationalOperator  Operator===  OutDataTypeStr=boolean  RndMeth=Simplest
  StAErrSet : Subsystem
  Triggered Subsystem1 : Subsystem  TreatAsAtomicUnit=on
  Triggered Subsystem2 : Subsystem  TreatAsAtomicUnit=on
  Triggered Subsystem3 : Subsystem  TreatAsAtomicUnit=on
  Triggered Subsystem4 : Subsystem  TreatAsAtomicUnit=on
  Triggered Subsystem5 : Subsystem  TreatAsAtomicUnit=on
  TM_St_Qis/w : Outport
  wires:
  Demux/2 -> Triggered Subsystem1/1(In1)
  Demux1/1 -> Relational Operator7/2, Relational Operator2/2
  Demux1/2 -> Triggered Subsystem2/1(In1)
  Demux2/1 -> Relational Operator8/2, Relational Operator3/2
  Demux3/1 -> Relational Operator9/2, Relational Operator4/2
  Demux3/2 -> Triggered Subsystem4/1(In1)
  TC_StErr_Constant/1 -> Demux/1
  TC_StErr_WildValue/1 -> Demux1/1
  TC_StErr_Fluctuation/1 -> Demux3/1
  Triggered Subsystem1/1(Out1) -> StAErrSet/2(TC_StErr_Constant)
  Triggered Subsystem2/1(Out1) -> StAErrSet/3(TC_StErr_WildValue)
  Triggered Subsystem3/1(Out1) -> StAErrSet/4(TC_StErr_Jump)
  Triggered Subsystem4/1(Out1) -> StAErrSet/5(TC_StErr_Wave)
  Demux4/1 -> If/1
  If/1 -> If Action Subsystem/Action
  Demux4/2 -> Quaternion Normalize/1
  If/2 -> If Action Subsystem1/Action
  StAErrSet/1(TM_St_Qis) -> If Action Subsystem1/1(In1)
  If Action Subsystem/1(Out1) -> Merge/1
  If Action Subsystem1/1(Out1) -> Merge/2
  Demux2/2 -> Triggered Subsystem3/1(In1)
  TC_StErr_Jump/1 -> Demux2/1
  Triggered Subsystem5/1(Out1) -> Demux4/1
  TC_StGNDSet/1 -> Demux5/1
  StNum/1 -> Relational Operator4/1, Relational Operator3/1, Relational Operator2/1, Relational Operator1/1, Relational Operator/1
  Relational Operator5/1 -> Logical Operator/1
  Demux5/1 -> Relational Operator5/2, Relational Operator/2
  Constant/1 -> Relational Operator5/1
  Relational Operator/1 -> Logical Operator/2
  Logical Operator/1 -> Triggered Subsystem5/Enable
  Relational Operator6/1 -> Logical Operator1/1
  Constant1/1 -> Relational Operator9/1, Relational Operator8/1, Relational Operator7/1, Relational Operator6/1
  Demux/1 -> Relational Operator6/2, Relational Operator1/2
  Relational Operator1/1 -> Logical Operator1/2
  Logical Operator1/1 -> Triggered Subsystem1/Enable
  Relational Operator2/1 -> Logical Operator2/2
  Logical Operator2/1 -> Triggered Subsystem2/Enable
  Relational Operator7/1 -> Logical Operator2/1
  Relational Operator3/1 -> Logical Operator3/2
  Logical Operator3/1 -> Triggered Subsystem3/Enable
  Relational Operator8/1 -> Logical Operator3/1
  Logical Operator4/1 -> Triggered Subsystem4/Enable
  Relational Operator4/1 -> Logical Operator4/2
  Relational Operator9/1 -> Logical Operator4/1
  Demux5/2 -> Triggered Subsystem5/1(In1)
  Quaternion Normalize/1 -> If Action Subsystem/1(In1)
  Merge/1 -> From Q to W/1(q), Mux/1
  From Q to W/1(w) -> Mux/2
  Mux/1 -> TM_St_Qis/w/1
  Qis_St/1 -> StAErrSet/1(Qis_St)

== system GS_model/Subsystem2/Subsystem/Sensor/StA&B&C&DModel1/StAMathModel2/StMathModel ==
  note: Qbs_St
  Qib : Inport
  Cons_StNoise : Inport  Port=2
  Qsb_StFix : Inport  Port=3
  TC_StFixErr : Inport  Port=4
  TC_StNoiseCoff : Inport  Port=5
  StNum : Inport  Port=6
  3 : Subsystem
  Constant : Constant  Value=0
  Constant1 : Constant  Value=0
  Demux : Demux  Outputs=[1;4]
  Demux1 : Demux  Outputs=2
  Logical Operator : Logic  Operator=OR  AllPortsSameDT=off  OutDataTypeStr=boolean
  Logical Operator1 : Logic  Operator=OR  AllPortsSameDT=off  OutDataTypeStr=boolean
  Quaternion Inverse : aerolibutil/Quaternion Inverse
  Quaternion Multiplication : aerolibutil/Quaternion Multiplication
  Quaternion Multiplication2 : aerolibutil/Quaternion Multiplication
  Quaternion Multiplication4 : aerolibutil/Quaternion Multiplication
  Quaternion Normalize : sharedutil/Quaternion Normalize  aMode=aMode
      settings: SourceProductBaseCode=AE,PW,MT,VE,VP
  Quaternion Normalize2 : sharedutil/Quaternion Normalize  aMode=aMode
      settings: SourceProductBaseCode=AE,PW,MT,VE,VP
  Relational Operator{,1..3} (4 alike) : RelationalOperator  Operator===  OutDataTypeStr=boolean  RndMeth=Simplest
  Triggered Subsystem1 : Subsystem  TreatAsAtomicUnit=on
  Triggered Subsystem2 : Subsystem  TreatAsAtomicUnit=on
  Qis_St : Outport
  wires:
  Triggered Subsystem2/1(Out1) -> 3/1(TC_StNoiseCoff)
  Demux/2 -> Triggered Subsystem1/1(In1)
  Triggered Subsystem1/1(Out1) -> Quaternion Normalize2/1
  Quaternion Normalize/1 -> Quaternion Multiplication/1
  Demux1/1 -> Relational Operator3/2, Relational Operator/2
  Demux1/2 -> Triggered Subsystem2/1(In1)
  Demux/1 -> Relational Operator2/2, Relational Operator1/2
  Quaternion Multiplication2/1 -> Quaternion Multiplication4/1
  TC_StNoiseCoff/1 -> Demux1/1
  Quaternion Normalize2/1 -> Quaternion Multiplication/2
  3/1(Q_StNoise) -> Quaternion Multiplication4/2
  Quaternion Multiplication/1 -> Quaternion Inverse/1
  Qib/1 -> Quaternion Multiplication2/1
  Qsb_StFix/1 -> Quaternion Normalize/1
  TC_StFixErr/1 -> Demux/1
  Quaternion Multiplication4/1 -> Qis_St/1
  Cons_StNoise/1 -> 3/2(Cons_StNoise)
  StNum/1 -> Relational Operator/1, Relational Operator1/1
  Relational Operator1/1 -> Logical Operator/2
  Constant/1 -> Relational Operator2/1
  Relational Operator2/1 -> Logical Operator/1
  Logical Operator/1 -> Triggered Subsystem1/Enable
  Relational Operator/1 -> Logical Operator1/2
  Constant1/1 -> Relational Operator3/1
  Relational Operator3/1 -> Logical Operator1/1
  Logical Operator1/1 -> Triggered Subsystem2/Enable
  Quaternion Inverse/1 -> Quaternion Multiplication2/2

== system GS_model/Subsystem2/Subsystem/Sensor/StA&B&C&DModel1/StAMathModel2/Subsystem ==
  note: 0-自主
      | 1-常有效
      | 2-常无效
  Sun_b : Inport
  Sunshine : Inport  Port=2
  Tc_ValidSet : Inport  Port=3
  Qsb_StAFix : Inport  Port=4
  SEA : Inport  Port=5
  EEA : Inport  Port=6
  Qob : Inport  Port=7
  Qis : Inport  Port=8
  StNum : Inport  Port=9
  Constant1 : Constant  Value=0
  Constant2 : Constant  Value=[1;0;0;0]
  Constant3 : Constant
  Constant4 : Constant  Value=0
  Demux1 : Demux  Outputs=2
  Logical Operator1 : Logic  Operator=OR  AllPortsSameDT=off  OutDataTypeStr=boolean
  Relational Operator : RelationalOperator  Operator===  OutDataTypeStr=boolean  RndMeth=Simplest
  Relational Operator3 : RelationalOperator  Operator===  OutDataTypeStr=boolean  RndMeth=Simplest
  Subsystem : Subsystem
  Switch : Switch  Criteria=u2 > Threshold  Threshold=0.5
  Switch1 : Switch  Criteria=u2 > Threshold  Threshold=0.5
  Switch2 : Switch  Criteria=u2 > Threshold  Threshold=1.5
  Triggered Subsystem2 : Subsystem  TreatAsAtomicUnit=on
  Agl_St&SunEarth : Outport
  Valid : Outport  Port=2
  Qis_St : Outport  Port=3
  wires:
  Switch/1 -> Qis_St/1
  Switch2/1 -> Valid/1, Switch/2
  Sun_b/1 -> Subsystem/1(Sun_b)
  Sunshine/1 -> Subsystem/2(Sunshine)
  Qsb_StAFix/1 -> Subsystem/3(Qsb_StAFix)
  SEA/1 -> Subsystem/4(SEA)
  EEA/1 -> Subsystem/5(EEA)
  Qob/1 -> Subsystem/6(Qob)
  Subsystem/2(Agl_St&SunEarth) -> Agl_St&SunEarth/1
  Relational Operator3/1 -> Logical Operator1/1
  Relational Operator/1 -> Logical Operator1/2
  Constant1/1 -> Relational Operator3/1
  Demux1/2 -> Triggered Subsystem2/1(In1)
  StNum/1 -> Relational Operator/1
  Demux1/1 -> Relational Operator3/2, Relational Operator/2
  Tc_ValidSet/1 -> Demux1/1
  Triggered Subsystem2/1(Out1) -> Switch1/2, Switch2/2
  Subsystem/1(Valid) -> Switch1/3
  Constant3/1 -> Switch1/1
  Switch1/1 -> Switch2/3
  Constant4/1 -> Switch2/1
  Logical Operator1/1 -> Triggered Subsystem2/Enable
  Qis/1 -> Switch/1
  Constant2/1 -> Switch/3

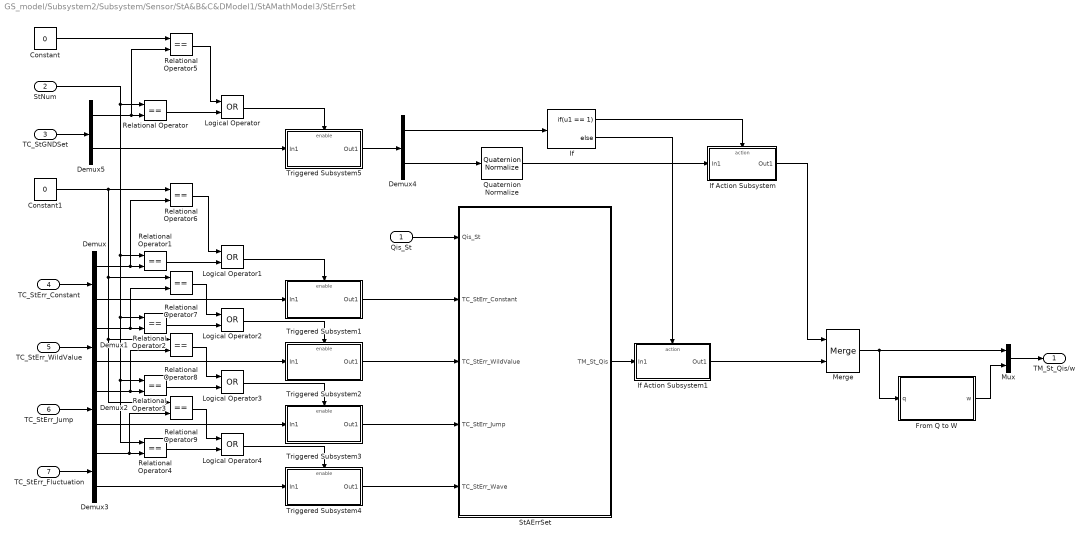
== system GS_model/Subsystem2/Subsystem/Sensor/StA&B&C&DModel1/StAMathModel3/StErrSet ==
  Qis_St : Inport
  StNum : Inport  Port=2
  TC_StGNDSet : Inport  Port=3
  TC_StErr_Constant : Inport  Port=4
  TC_StErr_WildValue : Inport  Port=5
  TC_StErr_Jump : Inport  Port=6
  TC_StErr_Fluctuation : Inport  Port=7
  Constant : Constant  Value=0
  Constant1 : Constant  Value=0
  Demux : Demux  Outputs=2
  Demux1 : Demux  Outputs=2
  Demux2 : Demux  Outputs=[1;3]
  Demux3 : Demux  Outputs=[1;2]
  Demux4 : Demux  Outputs=[1;4]
  Demux5 : Demux  Outputs=[1;5]
  From Q to W : Subsystem
  If : If  IfExpression=u1 == 1
  If Action Subsystem : Subsystem  TreatAsAtomicUnit=on
  If Action Subsystem1 : Subsystem  TreatAsAtomicUnit=on
  Logical Operator{,1..4} (5 alike) : Logic  Operator=OR  AllPortsSameDT=off  OutDataTypeStr=boolean
  Merge : Merge
  Mux : Mux  Inputs=2
  Quaternion Normalize : sharedutil/Quaternion Normalize  aMode=aMode
      settings: SourceProductBaseCode=AE,PW,MT,VE,VP
  Relational Operator{,1..9} (10 alike) : RelationalOperator  Operator===  OutDataTypeStr=boolean  RndMeth=Simplest
  StAErrSet : Subsystem
  Triggered Subsystem1 : Subsystem  TreatAsAtomicUnit=on
  Triggered Subsystem2 : Subsystem  TreatAsAtomicUnit=on
  Triggered Subsystem3 : Subsystem  TreatAsAtomicUnit=on
  Triggered Subsystem4 : Subsystem  TreatAsAtomicUnit=on
  Triggered Subsystem5 : Subsystem  TreatAsAtomicUnit=on
  TM_St_Qis/w : Outport
  wires:
  Qis_St/1 -> StAErrSet/1(Qis_St)
  Mux/1 -> TM_St_Qis/w/1
  From Q to W/1(w) -> Mux/2
  Merge/1 -> Mux/1, From Q to W/1(q)
  Quaternion Normalize/1 -> If Action Subsystem/1(In1)
  Demux5/2 -> Triggered Subsystem5/1(In1)
  Relational Operator9/1 -> Logical Operator4/1
  Relational Operator4/1 -> Logical Operator4/2
  Logical Operator4/1 -> Triggered Subsystem4/Enable
  Relational Operator8/1 -> Logical Operator3/1
  Logical Operator3/1 -> Triggered Subsystem3/Enable
  Relational Operator3/1 -> Logical Operator3/2
  Relational Operator7/1 -> Logical Operator2/1
  Logical Operator2/1 -> Triggered Subsystem2/Enable
  Relational Operator2/1 -> Logical Operator2/2
  Logical Operator1/1 -> Triggered Subsystem1/Enable
  Relational Operator1/1 -> Logical Operator1/2
  Demux/1 -> Relational Operator1/2, Relational Operator6/2
  Constant1/1 -> Relational Operator6/1, Relational Operator7/1, Relational Operator8/1, Relational Operator9/1
  Relational Operator6/1 -> Logical Operator1/1
  Logical Operator/1 -> Triggered Subsystem5/Enable
  Relational Operator/1 -> Logical Operator/2
  Constant/1 -> Relational Operator5/1
  Demux5/1 -> Relational Operator/2, Relational Operator5/2
  Relational Operator5/1 -> Logical Operator/1
  StNum/1 -> Relational Operator/1, Relational Operator1/1, Relational Operator2/1, Relational Operator3/1, Relational Operator4/1
  TC_StGNDSet/1 -> Demux5/1
  Triggered Subsystem5/1(Out1) -> Demux4/1
  TC_StErr_Jump/1 -> Demux2/1
  Demux2/2 -> Triggered Subsystem3/1(In1)
  If Action Subsystem1/1(Out1) -> Merge/2
  If Action Subsystem/1(Out1) -> Merge/1
  StAErrSet/1(TM_St_Qis) -> If Action Subsystem1/1(In1)
  If/2 -> If Action Subsystem1/Action
  Demux4/2 -> Quaternion Normalize/1
  If/1 -> If Action Subsystem/Action
  Demux4/1 -> If/1
  Triggered Subsystem4/1(Out1) -> StAErrSet/5(TC_StErr_Wave)
  Triggered Subsystem3/1(Out1) -> StAErrSet/4(TC_StErr_Jump)
  Triggered Subsystem2/1(Out1) -> StAErrSet/3(TC_StErr_WildValue)
  Triggered Subsystem1/1(Out1) -> StAErrSet/2(TC_StErr_Constant)
  TC_StErr_Fluctuation/1 -> Demux3/1
  TC_StErr_WildValue/1 -> Demux1/1
  TC_StErr_Constant/1 -> Demux/1
  Demux3/2 -> Triggered Subsystem4/1(In1)
  Demux3/1 -> Relational Operator4/2, Relational Operator9/2
  Demux2/1 -> Relational Operator3/2, Relational Operator8/2
  Demux1/2 -> Triggered Subsystem2/1(In1)
  Demux1/1 -> Relational Operator2/2, Relational Operator7/2
  Demux/2 -> Triggered Subsystem1/1(In1)
